simulink model "LQR_c_2015a"  (R2015a)
settings: Solver=ode4  SolverMode=SingleTasking  StartTime=0.0  StopTime=10  FixedStep=8e-5  RelTol=1e-3
values from neighbouring files (symbols this model uses):
  LQRopt = lqrd(A,B,Q,R,8e-5)    [initParams.m]    (also in teste.m)
settings Model: CovMetricSettings=dwe  CovHtmlReporting=off  covSaveCumulativeToWorkspaceVar=off  CovSaveSingleToWorkspaceVar=off  CovExternalEMLEnable=on  Creator=seumagal  LastModifiedBy=zoero
settings DataIOCC: LimitDataPoints=off  SaveFormat=Dataset
settings DebuggingCC: SFUnexpectedBacktrackingDiag=error  SFNoUnconditionalDefaultTransitionDiag=error
settings HardwareCC: ProdBitPerPointer=64  ProdLargestAtomicFloat=Float  ProdIntDivRoundTo=Zero  ProdEndianess=LittleEndian  ProdHWDeviceType=Specified
settings ModelReferenceCC: PropagateSignalLabelsOutOfModel=on
settings GRTTargetCC: TargetLangStandard=C99 (ISO)

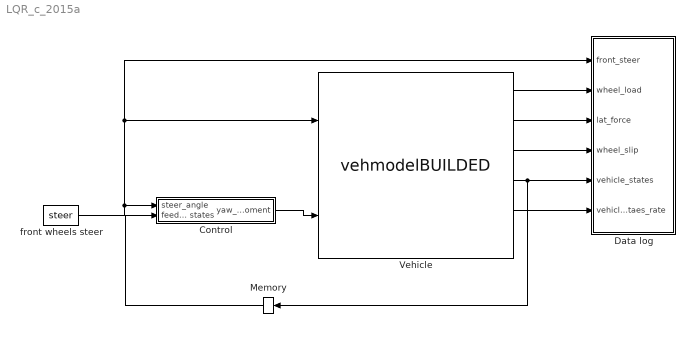
== system LQR_c_2015a ==
  "Control " : Subsystem  TreatAsAtomicUnit=on
  Data log : Subsystem
  Memory : Memory  X0=[0,80/3.6,0,0,0]
  Vehicle : S-Function  InitFcn=try, set_param(gcb,'FunctionName','vehmodelBUILDED'), end  FunctionName=vehmodelBUILDED  Parameters=params  SFunctionModules=vehmodelBUILDED_wrapper  mask(S-Function Builder){}
      mask help: Simulink:masks:SFunctionBuilder_MD
      mask init:
      | val = [[.9  0.75 0.75 1 1 .9 .9 1]',[1 1 0.75 0.75 .9 .9 1 .9]'];try , sys = get_param(gcb,'SfunBuilderFcnName');if isempty(sys), sys = get_param(gcb,'FunctionName'); end,catch, sys = get_param(gcb,'FunctionName'); end
      settings: CopyFcn=set_param(gcbh,'LinkStatus','none')  PreSaveFcn=try, set_param(gcb,'FunctionName','vehmodelBUILDED'), end  OpenFcn=sfunctionwizard(gcbh)
      mask Display: plot(val(:,1),val(:,2)),disp(sys), port_label('input',1,'inSteer'), port_label('input',2,'inMz'), port_label('output',1,'outFz'), port_label('output',2,'outFy'), port_label('output',3,'outSlip'), port_label('output',4,'outStates'), port_label('output',5,'outDStates')
  front wheels steer : FromWorkspace  VariableName=steer  SampleTime=0
  wires:
  front wheels steer/1 -> Data log/1(front_steer), Vehicle/1, "Control "/1(steer_angle)
  "Control "/1(yaw_moment) -> Vehicle/2
  Memory/1 -> "Control "/2(feedback states)
  Vehicle/1 -> Data log/2(wheel_load)
  Vehicle/2 -> Data log/3(lat_force)
  Vehicle/3 -> Data log/4(wheel_slip)
  Vehicle/4 -> Memory/1, Data log/5(vehicle_states)
  Vehicle/5 -> Data log/6(vehicle_staes_rate)

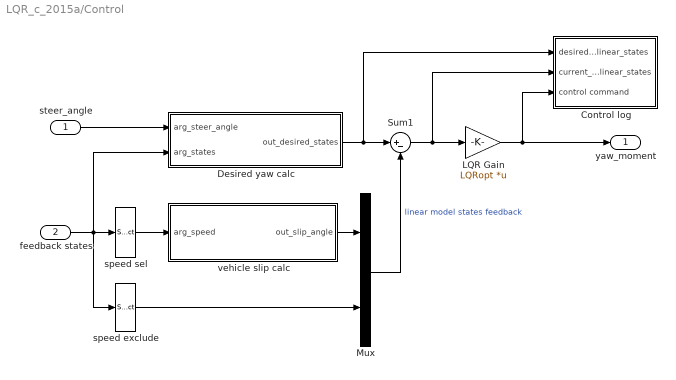
== system LQR_c_2015a/Control  ==
  steer_angle : Inport
  feedback states : Inport  Port=2
  Control log : Subsystem
  Desired yaw calc : MATLAB Function  TreatAsAtomicUnit=on
  LQR Gain : Gain  Gain=LQRopt  Multiplication=Matrix(K*u)
  Mux : Mux  Inputs=2
  Sum1 : Sum  Inputs=|+-
  "speed exclude " : Selector  InputPortWidth=5  Indices=[3,4,5]
  speed sel : Selector  InputPortWidth=5  Indices=[1,2]
  vehicle slip calc : MATLAB Function  TreatAsAtomicUnit=on
  yaw_moment : Outport
  wires:
  LQR Gain/1 -> yaw_moment/1, Control log/3(control command)
  steer_angle/1 -> Desired yaw calc/1(arg_steer_angle)
  Desired yaw calc/1(out_desired_states) -> Sum1/1, Control log/1(desired_linear_states)
  feedback states/1 -> Desired yaw calc/2(arg_states), "speed exclude "/1, speed sel/1
  vehicle slip calc/1(out_slip_angle) -> Mux/1
  speed sel/1 -> vehicle slip calc/1(arg_speed)
  Mux/1 -> Sum1/2  "linear model states feedback"
  "speed exclude "/1 -> Mux/2
  Sum1/1 -> LQR Gain/1, Control log/2(current_linear_states)

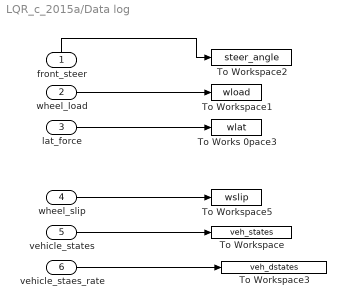
== system LQR_c_2015a/Data log ==
  front_steer : Inport
  wheel_load : Inport  Port=2
  lat_force : Inport  Port=3
  wheel_slip : Inport  Port=4
  vehicle_states : Inport  Port=5
  vehicle_staes_rate : Inport  Port=6
  To Works 0pace3 : ToWorkspace  VariableName=wlat  SaveFormat=Timeseries  SampleTime=-1
  To Workspace : ToWorkspace  VariableName=veh_states  SaveFormat=Timeseries  SampleTime=-1
  To Workspace1 : ToWorkspace  VariableName=wload  SaveFormat=Timeseries  SampleTime=-1
  To Workspace2 : ToWorkspace  VariableName=steer_angle  SaveFormat=Timeseries  SampleTime=-1
  To Workspace3 : ToWorkspace  VariableName=veh_dstates  SaveFormat=Timeseries  SampleTime=-1
  To Workspace5 : ToWorkspace  VariableName=wslip  SaveFormat=Timeseries  SampleTime=-1
  wires:
  lat_force/1 -> To Works 0pace3/1
  wheel_load/1 -> To Workspace1/1
  vehicle_staes_rate/1 -> To Workspace3/1
  wheel_slip/1 -> To Workspace5/1
  vehicle_states/1 -> To Workspace/1
  front_steer/1 -> To Workspace2/1

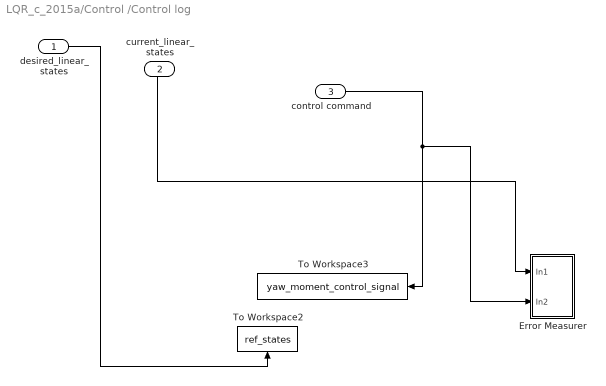
== system LQR_c_2015a/Control /Control log ==
  desired_linear_states : Inport
  current_linear_states : Inport  Port=2
  control command : Inport  Port=3
  Error Measurer : Subsystem
  To Workspace2 : ToWorkspace  VariableName=ref_states  SaveFormat=Timeseries  SampleTime=-1
      settings: MaxDataPoints=Inf
  To Workspace3 : ToWorkspace  VariableName=yaw_moment_control_signal  SaveFormat=Timeseries  SampleTime=-1
      settings: MaxDataPoints=Inf
  wires:
  current_linear_states/1 -> Error Measurer/1(In1)
  control command/1 -> To Workspace3/1, Error Measurer/2(In2)
  desired_linear_states/1 -> To Workspace2/1

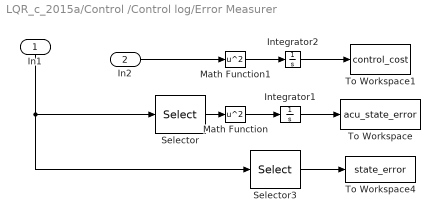
== system LQR_c_2015a/Control /Control log/Error Measurer ==
  In1 : Inport
  In2 : Inport  Port=2
  Integrator1 : Integrator
  Integrator2 : Integrator
  Math Function : Math  Operator=square  SaturateOnIntegerOverflow=on
  Math Function1 : Math  Operator=square  SaturateOnIntegerOverflow=on
  Selector : Selector  InputPortWidth=4  Indices=[1 2]
  Selector3 : Selector  InputPortWidth=4  Indices=[1 2]
  To Workspace : ToWorkspace  VariableName=acu_state_error  SaveFormat=Timeseries  SampleTime=-1
      settings: MaxDataPoints=1
  To Workspace1 : ToWorkspace  VariableName=control_cost  SaveFormat=Timeseries  SampleTime=-1
      settings: MaxDataPoints=1
  To Workspace4 : ToWorkspace  VariableName=state_error  SaveFormat=Timeseries  SampleTime=-1
      settings: MaxDataPoints=Inf
  wires:
  In1/1 -> Selector3/1, Selector/1
  In2/1 -> Math Function1/1
  Integrator1/1 -> To Workspace/1
  Math Function1/1 -> Integrator2/1
  Math Function/1 -> Integrator1/1
  Integrator2/1 -> To Workspace1/1
  Selector/1 -> Math Function/1
  Selector3/1 -> To Workspace4/1

== matlab function LQR_c_2015a/Control /vehicle slip calc ==
  data: arg_speed input; out_slip_angle output
function out_slip_angle = slipangle(arg_speed)

out_slip_angle = atan2(arg_speed(1),arg_speed(2));

== matlab function LQR_c_2015a/Control /Desired yaw calc ==
  data: arg_steer_angle input; out_desired_states output; arg_states input
function out_desired_states  = desired_states( arg_steer_angle, arg_states )

persistent mu_g;
persistent Ku;
persistent l;

if isempty(Ku)
    modelParams = coder.load( 'modelParam.mat' );
    mu_g = modelParams.friction_coefficient*modelParams.g;
    l = modelParams.l;
    Ku = modelParams.Ku;
end

long_speed = arg_states(2);
aux = (l + Ku*long_speed*long_speed);
desired_yaw_rate = long_speed*arg_steer_angle/aux;


desired_yaw_rate = min([abs(desired_yaw_rate), abs(mu_g/long_speed)])*sign(arg_steer_angle);

%desired_slip = atan2(arg_states(1),arg_states(2));
%if abs(desired_slip) > (10*pi/180) 
%    desired_slip = 10*pi/180*sign(desired_slip);
%end

out_desired_states = [0; desired_yaw_rate; 0; 0 ];

end
